simulink model "concept3_simulink_RL"  (R2025a)
settings: Solver=VariableStepAuto  StartTime=0.0  StopTime=Tf  FixedStep=0.001  MaxStep=0.01  MinStep=0.0001  RelTol=1e-3
InitFcn:
  | loaded_data = load('concept3_for_sim.mat');
  | robot = loaded_data.robot;
  | robot.DataFormat = 'column';
values from neighbouring files (symbols this model uses):
  mass = 40    [RL_main.m]    (also in baseline_sim.m)
  obs_vec = opa    [RL_main.m]    (also in baseline_sim.m)
  port = data(n, :)    [RL_main.m]    (also in baseline_sim.m = port_pos_data(n,:))
  port_num = 10    [RL_main.m]    (also in baseline_sim.m)
  port_target = AB2port(port_num)    [RL_main.m]    (also in baseline_sim.m)
  q0arm = rad2deg([-1.283; -1.622; 2.2761853; -1.8021853; 1.112; 1.859; 0.05328])    [RL_main.m]    (also in baseline_sim.m)
  q0b = [1; 0; 0; 0; 0; 0; 0]    [RL_main.m]    (also in baseline_sim.m = [1;0;0;0;0;0;0])
  sat_docked = AB2port(sat_docked_num)    [RL_main.m]    (also in baseline_sim.m)
  sat_docked_num = 6    [RL_main.m]    (also in baseline_sim.m)
  sim_state = 1    [RL_main.m]    (also in baseline_sim.m)
  Tlog = 0.1    [RL_main.m]    (also in baseline_sim.m)
  use_RL = 1    [RL_main.m]    (also in baseline_sim.m)
undefined symbols (not defined in the file or in its folder): opa, target, X, Y, Z
libraries: sm_lib x133, nesl_utility x67, simulink_extras x3, rllib x2
(part 5 of 6)

== matlab function concept3_simulink_RL/QP1/MATLAB Function2 ==
  data: ydot output; y output; done output; clock input; fromPort input; toPort input; seg output
function [ydot, y, done, seg] = Poly_traj_selector(clock, fromPort, toPort)
%#codegen
% Poly_traj_selector
% 입력:
%   - clock [s] : Simulink Clock 출력
%   - fromPort  : 시작 포트 번호 (uint8/uint16 권장)
%   - toPort    : 도착 포트 번호
%
% 출력:
%   - y = [x; y; z; roll; pitch; yaw] (deg for RPY)
%
% 설명:
% - 경로(포트쌍)별로 세그먼트 시간 T와 5차 다항 계수 coeffs를 등록해 둡니다.
% - 각 세그먼트는 정지/가속도0 경계조건을 만족하는 5차 다항 (열: [a5 a4 a3 a2 a1 a0]).
% - 세그먼트 개수는 예시로 3개(maxSeg=3)로 고정. (모자라면 뒤는 0초/0계수로 패딩)
% - 마지막 세그먼트 종료 이후에는 최종 자세를 홀드합니다.

% ===== 고정 파라미터 =====
maxSeg = int32(4);          % int32로 고정
nDOF   = int32(6);          % int32로 고정

% ===== 입력 포트 형 변환(내부는 int32 사용) =====
fromP = int32(fromPort);
toP   = int32(toPort);

% ===== 선택 키 (예: 6->10 = 610) =====
key = fromP*int32(100) + toP;

% ===== 메모리 미리 할당 (double) =====
T      = zeros(1, double(maxSeg));                % double
coeffs = zeros(double(nDOF), 6, double(maxSeg), 'like', clock);  % double
y      = zeros(double(nDOF), 1, 'like', clock);   % double
ydot   = zeros(double(nDOF), 1, 'like', clock);   % double
done = false;

switch key


    case 602
        % --- segment durations ---
        T1 = 47.987;
        T2 = 28;
        T3 = 20;
        T4 = 25;
        T  = [T1, T2, T3,T4];

        % --- coeffs(6,6,seg): rows=DOF [x y z roll pitch yaw], cols=[a5 a4 a3 a2 a1 a0] ---
        % Segment 1
        coeffs(:,:,1) = [ ...
 0	-0	 0	 0	 0	 2.5;
-3.18313416839e-08	 3.81874771732e-06	-0.000122167510444	 0	 0	 0.35;
 1.17893858088e-08	-1.41435100642e-06	 4.52472260904e-05	 0	 0	 0;
 0	-0	 0	 0	 0	-90;
 0	-0	 0	 0	 0	 0;
 0	-0	 0	 0	 0	-90

        ];

        % Segment 2
        coeffs(:,:,2) = [ ...
-4.88077884215e-07	 3.4165451895e-05	-0.000637755102041	 0	 0	 2.5;
 0	-0	 0	 0	 0	-1;
 0	-0	 0	 0	 0	 0.5;
 0	-0	 0	 0	 0	-90;
 0	-0	 0	 0	 0	 0;
 0	-0	 0	 0	 0	-90
        ];

        % Segment 3
        coeffs(:,:,3) = [ ...
 0	-0	 0	 0	 0	 1.1;
 0	-0	 0	 0	 0	-1;
 0	-0	 0	 0	 0	 0.5;
 0	-0	 0	 0	 0	-90;
 0	-0	 0	 0	 0	 0;
-0.00016875	 0.0084375	-0.1125	 0	 0	-90
        ];


        % Segment 4
        coeffs(:,:,4) = [ ...
 0	-0	 0	 0	 0	 1.1;
 0	-0	 0	 0	 0	-1;
-3.072e-07	 1.92e-05	-0.00032	 0	 0	 0.5;
 0	-0	 0	 0	 0	-90;
 0	-0	 0	 0	 0	 0;
 0	-0	 0	 0	 0	-180
        ];



 case 603
        % --- segment durations ---
        T1 = 47.987;
        T2 = 38;
        T3 = 20.0;
        T4 = 25;
        T  = [T1, T2, T3, T4];

        % --- coeffs(6,6,seg): rows=DOF [x y z roll pitch yaw], cols=[a5 a4 a3 a2 a1 a0] ---
        % Segment 1
        coeffs(:,:,1) = [ ...
 0	-0	 0	 0	 0	 2.5;
-3.18313416839e-08	 3.81874771732e-06	-0.000122167510444	 0	 0	 0.35;
 1.17893858088e-08	-1.41435100642e-06	 4.52472260904e-05	 0	 0	 0;
 0	-0	 0	 0	 0	-90;
 0	-0	 0	 0	 0	 0;
 0	-0	 0	 0	 0	-90
        ];

        % Segment 2
        coeffs(:,:,2) = [ ...
-1.43875507401e-07	 1.36681732031e-05	-0.000346260387812	 0	 0	 2.5;
 0	-0	 0	 0	 0	-1;
 0	-0	 0	 0	 0	 0.5;
 0	-0	 0	 0	 0	-90;
 0	-0	 0	 0	 0	 0;
 0	-0	 0	 0	 0	-90
        ];

        % Segment 3
        coeffs(:,:,3) = [ ...
 0	-0	 0	 0	 0	 0.6;
 0	-0	 0	 0	 0	-1;
 0	-0	 0	 0	 0	 0.5;
 0	-0	 0	 0	 0	-90;
 0	-0	 0	 0	 0	 0;
-0.00016875	 0.0084375	-0.1125	 0	 0	-90
        ];


        % Segment 4
        coeffs(:,:,4) = [ ...
 0	-0	 0	 0	 0	 0.6;
 0	-0	 0	 0	 0	-1;
-3.072e-07	 1.92e-05	-0.00032	 0	 0	 0.5;
 0	-0	 0	 0	 0	-90;
 0	-0	 0	 0	 0	 0;
 0	-0	 0	 0	 0	-180
        ];

    case 604
        % --- segment durations ---
        T1 = 47.987;
        T2 = 48;
        T3 = 20.0;
        T4 = 25;
        T  = [T1, T2, T3, T4];

        % --- coeffs(6,6,seg): rows=DOF [x y z roll pitch yaw], cols=[a5 a4 a3 a2 a1 a0] ---
        % Segment 1
        coeffs(:,:,1) = [ ...;
 0	-0	 0	 0	 0	 2.5;
-3.18313416839e-08	 3.81874771732e-06	-0.000122167510444	 0	 0	 0.35;
 1.17893858088e-08	-1.41435100642e-06	 4.52472260904e-05	 0	 0	 0;
 0	-0	 0	 0	 0	-90;
 0	-0	 0	 0	 0	 0;
 0	-0	 0	 0	 0	-90
        ];

        % Segment 2
        coeffs(:,:,2) = [ ...
-5.65140335648e-08	 6.78168402778e-06	-0.000217013888889	 0	 0	 2.5;
 0	-0	 0	 0	 0	-1;
 0	-0	 0	 0	 0	 0.5;
 0	-0	 0	 0	 0	-90;
 0	-0	 0	 0	 0	 0;
 0	-0	 0	 0	 0	-90
        ];

        % Segment 3
        coeffs(:,:,3) = [ ...
 0	-0	 0	 0	 0	 0.1;
 0	-0	 0	 0	 0	-1;
 0	-0	 0	 0	 0	 0.5;
 0	-0	 0	 0	 0	-90;
 0	-0	 0	 0	 0	 0;
-0.00016875	 0.0084375	-0.1125	 0	 0	-90
        ];

        % Segment 4
        coeffs(:,:,4) = [ ...
 0	-0	 0	 0	 0	 0.1;
 0	-0	 0	 0	 0	-1;
-3.072e-07	 1.92e-05	-0.00032	 0	 0	 0.5;
 0	-0	 0	 0	 0	-90;
 0	-0	 0	 0	 0	 0;
 0	-0	 0	 0	 0	-180
        ];


    case 605
        % --- segment durations ---
        T1 = 47.987;
        T2 = 58.000;
        T3 = 20;
        T4 = 25;
        T  = [T1, T2, T3, T4];

        % --- coeffs(6,6,seg): rows=DOF [x y z roll pitch yaw], cols=[a5 a4 a3 a2 a1 a0] ---
        % Segment 1
        coeffs(:,:,1) = [ ...;
 0	-0	 0	 0	 0	 2.5;
-3.18313416839e-08	 3.81874771732e-06	-0.000122167510444	 0	 0	 0.35;
 1.17893858088e-08	-1.41435100642e-06	 4.52472260904e-05	 0	 0	 0;
 0	-0	 0	 0	 0	-90;
 0	-0	 0	 0	 0	 0;
 0	-0	 0	 0	 0	-90
        ];

        % Segment 2
        coeffs(:,:,2) = [ ...
-2.65099726983e-08	 3.84394604125e-06	-0.000148632580262	 0	 0	 2.5;
 0	-0	 0	 0	 0	-1;
 0	-0	 0	 0	 0	 0.5;
 0	-0	 0	 0	 0	-90;
 0	-0	 0	 0	 0	 0;
 0	-0	 0	 0	 0	-90
        ];

        % Segment 3
        coeffs(:,:,3) = [ ...
 0	-0	 0	 0	 0	-0.4;
 0	-0	 0	 0	 0	-1;
 0	-0	 0	 0	 0	 0.5;
 0	-0	 0	 0	 0	-90;
 0	-0	 0	 0	 0	 0;
-0.00016875	 0.0084375	-0.1125	 0	 0	-90
        ];

        % Segment 4
        coeffs(:,:,4) = [ ...
 0	-0	 0	 0	 0	-0.4;
 0	-0	 0	 0	 0	-1;
-3.072e-07	 1.92e-05	-0.00032	 0	 0	 0.5;
 0	-0	 0	 0	 0	-90;
 0	-0	 0	 0	 0	 0;
 0	-0	 0	 0	 0	-180
        ];

    case 607
        % --- segment durations ---
        T1 = 27.335;
        T2 = 28.;
        T3 = 20;
        T4 = 25;
        T  = [T1, T2, T3,T4];

        % --- coeffs(6,6,seg): rows=DOF [x y z roll pitch yaw], cols=[a5 a4 a3 a2 a1 a0] ---
        % Segment 1
        coeffs(:,:,1) = [ ...
 0	-0	 0	 0	 0	 2.5;
 2.55528978563e-07	-1.74624452398e-05	 0.000318228218674	 0	 0	 0.35;
 1.96560752741e-07	-1.34326501845e-05	 0.000244790937442	 0	 0	 0;
 0	-0	 0	 0	 0	-90;
 0	-0	 0	 0	 0	 0;
 0	-0	 0	 0	 0	-90
        ];

        % Segment 2
        coeffs(:,:,2) = [ ...
-4.88077884215e-07	 3.4165451895e-05	-0.000637755102041	 0	 0	 2.5;
 0	-0	 0	 0	 0	 1;
 0	-0	 0	 0	 0	 0.5;
 0	-0	 0	 0	 0	-90;
 0	-0	 0	 0	 0	 0;
 0	-0	 0	 0	 0	-90
        ];

        % Segment 3
        coeffs(:,:,3) = [ ...
 0	-0	 0	 0	 0	 1.1;
 0	-0	 0	 0	 0	 1;
 0	-0	 0	 0	 0	 0.5;
 0	-0	 0	 0	 0	-90;
 0	-0	 0	 0	 0	 0;
 0.00016875	-0.0084375	 0.1125	 0	 0	-90
        ];

                % Segment 4
        coeffs(:,:,4) = [ ...
 0	-0	 0	 0	 0	 1.1;
 0	-0	 0	 0	 0	 1;
-3.072e-07	 1.92e-05	-0.00032	 0	 0	 0.5;
 0	-0	 0	 0	 0	-90;
 0	-0	 0	 0	 0	 0;
 0	-0	 0	 0	 0	 0
        ];

    case 608
        % --- segment durations ---
        T1 = 27.335;
        T2 = 38;
        T3 = 20;
        T4 = 25;
        T  = [T1, T2, T3,T4];

        % --- coeffs(6,6,seg): rows=DOF [x y z roll pitch yaw], cols=[a5 a4 a3 a2 a1 a0] ---
        % Segment 1
        coeffs(:,:,1) = [ ...
 0	-0	 0	 0	 0	 2.5;
 2.55528978563e-07	-1.74624452398e-05	 0.000318228218674	 0	 0	 0.35;
 1.96560752741e-07	-1.34326501845e-05	 0.000244790937442	 0	 0	 0;
 0	-0	 0	 0	 0	-90;
 0	-0	 0	 0	 0	 0;
 0	-0	 0	 0	 0	-90
        ];

        % Segment 2
        coeffs(:,:,2) = [ ...
-1.43875507401e-07	 1.36681732031e-05	-0.000346260387812	 0	 0	 2.5;
 0	-0	 0	 0	 0	 1;
 0	-0	 0	 0	 0	 0.5;
 0	-0	 0	 0	 0	-90;
 0	-0	 0	 0	 0	 0;
 0	-0	 0	 0	 0	-90
        ];

        % Segment 3
        coeffs(:,:,3) = [ ...
 0	-0	 0	 0	 0	 0.6;
 0	-0	 0	 0	 0	 1;
 0	-0	 0	 0	 0	 0.5;
 0	-0	 0	 0	 0	-90;
 0	-0	 0	 0	 0	 0;
 0.00016875	-0.0084375	 0.1125	 0	 0	-90

        ];

                % Segment 4
        coeffs(:,:,4) = [ ...
 0	-0	 0	 0	 0	 0.6;
 0	-0	 0	 0	 0	 1;
-3.072e-07	 1.92e-05	-0.00032	 0	 0	 0.5;
 0	-0	 0	 0	 0	-90;
 0	-0	 0	 0	 0	 0;
 0	-0	 0	 0	 0	 0
        ];
    
    case 609
        % --- segment durations ---
        T1 = 27.335;
        T2 = 48;
        T3 = 20;
        T4 = 25;
        T  = [T1, T2, T3, T4];

        % --- coeffs(6,6,seg): rows=DOF [x y z roll pitch yaw], cols=[a5 a4 a3 a2 a1 a0] ---
        % Segment 1
        coeffs(:,:,1) = [ ...
 0	-0	 0	 0	 0	 2.5;
 2.55528978563e-07	-1.74624452398e-05	 0.000318228218674	 0	 0	 0.35;
 1.96560752741e-07	-1.34326501845e-05	 0.000244790937442	 0	 0	 0;
 0	-0	 0	 0	 0	-90;
 0	-0	 0	 0	 0	 0;
 0	-0	 0	 0	 0	-90
        ];

        % Segment 2
        coeffs(:,:,2) = [ ...
-5.65140335648e-08	 6.78168402778e-06	-0.000217013888889	 0	 0	 2.5;
 0	-0	 0	 0	 0	 1;
 0	-0	 0	 0	 0	 0.5;
 0	-0	 0	 0	 0	-90;
 0	-0	 0	 0	 0	 0;
 0	-0	 0	 0	 0	-90
        ];

        % Segment 3
        coeffs(:,:,3) = [ ...
 0	-0	 0	 0	 0	 0.1;
 0	-0	 0	 0	 0	 1;
 0	-0	 0	 0	 0	 0.5;
 0	-0	 0	 0	 0	-90;
 0	-0	 0	 0	 0	 0;
 0.00016875	-0.0084375	 0.1125	 0	 0	-90
        ];

        % Segment 4
        coeffs(:,:,4) = [ ...
 0	-0	 0	 0	 0	 0.1;
 0	-0	 0	 0	 0	 1;
-3.072e-07	 1.92e-05	-0.00032	 0	 0	 0.5;
 0	-0	 0	 0	 0	-90;
 0	-0	 0	 0	 0	 0;
 0	-0	 0	 0	 0	 0
        ];
%{
%더 위로 많이 튀어오루는
 case 610
        % --- segment durations ---
        T1 = 34.359;
        T2 = 58.000;
        T3 = 20.0;
        T4 = 40.0;
        T  = [T1, T2, T3,T4];

        % --- coeffs(6,6,seg): rows=DOF [x y z roll pitch yaw], cols=[a5 a4 a3 a2 a1 a0] ---
        % Segment 1
        coeffs(:,:,1) = [ ...
 0	-0	 0	 0	 0	 2.5;
 8.14420194226e-08	-6.99570934256e-06	 0.000160244714142	 0	 0	 0.35;
 1.00236331597e-07	-8.61010380623e-06	 0.000197224263559	 0	 0	 0;
 0	-0	 0	 0	 0	-90;
 0	-0	 0	 0	 0	 0;
 0	-0	 0	 0	 0	-90
        ];

        % Segment 2
        coeffs(:,:,2) = [ ...
-2.65099726983e-08	 3.84394604125e-06	-0.000148632580262	 0	 0	 2.5;
 0	-0	 0	 0	 0	 1;
 0	-0	 0	 0	 0	 0.8;
 0	-0	 0	 0	 0	-90;
 0	-0	 0	 0	 0	 0;
 0	-0	 0	 0	 0	-90
        ];

        % Segment 3
        coeffs(:,:,3) = [ ...
 0	-0	 0	 0	 0	-0.4;
 0	-0	 0	 0	 0	 1;
 0	-0	 0	 0	 0	 0.8;
 0	-0	 0	 0	 0	-90;
 0	-0	 0	 0	 0	 0;
 0.00016875	-0.0084375	 0.1125	 0	 0	-90
        ];

        % Segment 4
        coeffs(:,:,4) = [ ...
 0	-0	 0	 0	 0	-0.4;
 0	-0	 0	 0	 0	 1;
-4.6875e-08	 4.6875e-06	-0.000125	 0	 0	 0.8;
 0	-0	 0	 0	 0	-90;
 0	-0	 0	 0	 0	 0;
 0	-0	 0	 0	 0	 0
        ];
%}


    case 610
        % --- segment durations ---
        T1 = 32.8718048721934 ;
        T2 = 58.000;
        T3 = 20.0;
        T4 = 26.9258240356725;
        T  = [T1, T2, T3,T4];

        % --- coeffs(6,6,seg): rows=DOF [x y z roll pitch yaw], cols=[a5 a4 a3 a2 a1 a0] ---
        % Segment 1
        coeffs(:,:,1) = [ ...
 0	-0	 0	 0	 0	 2.5;
 1.32877798661e-07	-1.09198326736e-05	 0.000239303072589	 0	 0	 0.35;
 7.81634109771e-08	-6.42343098446e-06	 0.000140766513288	 0	 0	 0;
 0	-0	 0	 0	 0	-90;
 0	-0	 0	 0	 0	 0;
 0	-0	 0	 0	 0	-90
        ];

        % Segment 2
        coeffs(:,:,2) = [ ...
-2.65099726983e-08	 3.84394604125e-06	-0.000148632580262	 0	 0	 2.5;
 0	-0	 0	 0	 0	 1.2;
 0	-0	 0	 0	 0	 0.5;
 0	-0	 0	 0	 0	-90;
 0	-0	 0	 0	 0	 0;
 0	-0	 0	 0	 0	-90
        ];

        % Segment 3
        coeffs(:,:,3) = [ ...
 0	-0	 0	 0	 0	-0.4;
 0	-0	 0	 0	 0	 1.2;
 0	-0	 0	 0	 0	 0.5;
 0	-0	 0	 0	 0	-90;
 0	-0	 0	 0	 0	 0;
 0.00016875	-0.0084375	 0.1125	 0	 0	-90
        ];

        % Segment 4
        coeffs(:,:,4) = [ ...
 0	-0	 0	 0	 0	-0.4;
-8.47883589298e-08	 5.70749108205e-06	-0.000102452600374	 0	 0	 1.2;
-2.11970897325e-07	 1.42687277051e-05	-0.000256131500934	 0	 0	 0.5;
 0	-0	 0	 0	 0	-90;
 0	-0	 0	 0	 0	 0;
 0	-0	 0	 0	 0	 0
        ];

        
    % =========================



    otherwise
        seg = double(0);
        return;
end
% ===== 누적 시간 & 세그먼트 선택(모두 int32 사용) =====
cumT = zeros(1, double(maxSeg));
cumT(1) = T(1);
for i = 2:double(maxSeg)
    cumT(i) = cumT(i-1) + T(i);
end

t = clock;
seg_i = int32(1);
t0 = 0.0;

% ===== 현재 세그먼트 판별 =====
if t <= 0
    seg_i = int32(1); t0 = 0.0;
else
    lastSeg = int32(1);
    for i = int32(1):maxSeg
        if T(double(i)) > 0
            lastSeg = i;
        end
    end

    if t < cumT(1)
        seg_i = int32(1); t0 = 0.0;
    elseif (maxSeg >= 2) && (T(2) > 0) && (t < cumT(2))
        seg_i = int32(2); t0 = cumT(1);
    elseif (maxSeg >= 3) && (T(3) > 0) && (t < cumT(3))
        seg_i = int32(3); t0 = cumT(2);
    elseif (maxSeg >= 4) && (T(4) > 0) && (t < cumT(4))
        seg_i = int32(4); t0 = cumT(3);
    else
        seg_i = lastSeg;
        if lastSeg == 1
            t0 = 0.0;
        else
            t0 = cumT(double(lastSeg-1));
        end
        t = cumT(double(lastSeg)); % clamp
        done = true;
    end
end

% ===== 현재 세그먼트 double로 변환해 출력용 저장 =====
seg = double(seg_i);

% ===== 세그먼트 상대시간 =====
tau = t - t0;

% ===== Horner 평가 =====
for d = 1:double(nDOF)
    a5 = coeffs(d,1,seg_i);
    a4 = coeffs(d,2,seg_i);
    a3 = coeffs(d,3,seg_i);
    a2 = coeffs(d,4,seg_i);
    a1 = coeffs(d,5,seg_i);
    a0 = coeffs(d,6,seg_i);
    y(d)    = ((((a5*tau + a4)*tau + a3)*tau + a2)*tau + a1)*tau + a0;
    ydot(d) = ((((5*a5*tau + 4*a4)*tau + 3*a3)*tau + 2*a2)*tau + a1);
end
ydot(4:6) = deg2rad(ydot(4:6));
%y(3) = 0;
%ydot(3) = 0;
end

== matlab function concept3_simulink_RL/R2L/obs ==
  data: q input; y output; qdot input; w_base input; Tau input; H_obs input; muRL input; sigmaRL input; muRL_new output; sigmaRL_new output
function [y, muRL_new, sigmaRL_new] = obs(q, qdot, w_base, Tau, H_obs, muRL, sigmaRL)
%% --------------------------------------------------------------
% q : [quat_base(4); basepos(3); joint(7)]  (14x1)
% qdot : (7x1)
% H_obs : RL_obs 벡터 (26x1)
% muRL, sigmaRL : 이전 호출의 통계량 (26x1)
% --------------------------------------------------------------
eps = 1e-8;
beta = 0.05;

%% (1) 입력 분리
qbase = q(1:4);
q_joint = q(8:14);

%% (2) 관절 각도/속도 정규화
q_min = [-1.3 -2.9 2.2 -2.8 1.1 1.3 0.1]';
q_max = [2.2 -1.6 4.4 -1.5 3.9 4.4 2.1]';
qdot_max = [0.2 0.07 0.1 0.08 0.23 0.1 0.08]';

q_mid = 0.5 * (q_max + q_min);
q_norm = 2 * (q_joint - q_mid) ./ (q_max - q_min);
qdot_norm = qdot ./ (qdot_max + eps);
qdot_norm = max(min(qdot_norm, 1), -1);

%% (3) 베이스 쿼터니언 정규화
q_base = qbase / (norm(qbase) + eps);   % 정규화
if q_base(1) < 0, q_base = -q_base; end % 연속성 확보

q_ref = [1;0;0;0];                      % 목표자세
q_err = quatmultiply(q_ref.', quatconj(q_base.')).';  % [w x y z]

if q_err(1) < 0, q_err = -q_err; end    % 부호 연속성

att_err_vec = 2 * q_err(2:4);
qbase = att_err_vec / deg2rad(20);   % 약 [-1,1] 범위로 정규화


%% 베이스 속도 정규화
qb_max = 0.004; qb_min = -0.004;
qb_mid = 0.5 * (qb_max + qb_min);
qb_norm = 2 * (w_base - qb_mid) ./ (qb_max - qb_min);

%% 토크 정규화
t_max = 3; t_min = -3;
t_mid = 0.5 * (t_max + t_min);
t_norm = 2 * (Tau - t_mid) ./ (t_max - t_min);

%% (4) RL_obs 정규화
RL_obs = H_obs(:);
RL_log = sign(RL_obs) .* log(1 + abs(RL_obs));

% 입력된 muRL, sigmaRL이 없으면 기본값 세팅
if isempty(muRL)
    muRL = zeros(size(RL_obs));
    sigmaRL = ones(size(RL_obs));
end

% 러닝 평균 갱신
muRL_new    = (1 - beta) * muRL + beta * RL_log;
sigmaRL_new = (1 - beta) * sigmaRL + beta * abs(RL_log - muRL_new);

% 정규화 및 클리핑
RL_norm = (RL_log - muRL_new) ./ (sigmaRL_new + eps);
RL_norm = max(min(RL_norm, 5), -5);

% RL_norm 빼면 18

%% (5) 출력 구성

%y = [q_norm; qdot_norm; qbase; qb_norm; t_norm; RL_norm];
y = [q_norm; qdot_norm; t_norm];
end

== matlab function concept3_simulink_RL/Plant/Docking logic/Docking sensor/Subsystem/Quat2RPY ==
  data: q_current input; RPY output
function RPY = fcn(q_current)

sequence = 'ZYX';

eul_angles_rad_out = quat2eul(q_current', sequence);

%eul_angles_deg_out = rad2deg(eul_angles_rad_out);

yaw_out = eul_angles_rad_out(1);
pitch_out = eul_angles_rad_out(2);
roll_out = eul_angles_rad_out(3);

RPY = [roll_out; pitch_out; yaw_out];

== matlab function concept3_simulink_RL/Plant/station_robot_arm/Subsystem/Quat2RPY ==
  data: q_current input; RPY output
function RPY = fcn(q_current)

sequence = 'ZYX';

eul_angles_rad_out = quat2eul(q_current', sequence);

eul_angles_deg_out = rad2deg(eul_angles_rad_out);

yaw_deg_out = eul_angles_deg_out(1);
pitch_deg_out = eul_angles_deg_out(2);
roll_deg_out = eul_angles_deg_out(3);

RPY = [roll_deg_out; pitch_deg_out; yaw_deg_out];

== matlab function concept3_simulink_RL/R2L/MATLAB Function1 ==
  data: xb_q input; w_base input; tau input; r output
function r = reward_fn(xb_q,w_base, tau)
%#codegen
% RL 보상함수 (exponential terminal shaping)
% xb_q : [quat(4); pos(3)]
% q : full state (joint 포함)
% tau : joint torque
% done : episode 종료 flag

%% ====== 가중치 설정 ======
alpha = 0.3;    % 조인트 복귀 가중치
beta  = 20000.0;    % 베이스 각속도
gamma = 200;     % 토크 절약 가중치
delta = 150;   % 베이스 자세 오차 가중치

offset = 0.0;     % baseline offset (critic 안정화용)
scale = 1;      % 전체 보상 스케일 조절

%% ====== 데이터 정리 ======
xb_q = double(xb_q(:));
%q    = double(q(:));
tau  = double(tau(:));
w_base = double(w_base(:));
k_att = 1.0;

%% ====== (1) 조인트각 오차 ======
%{
qhome = deg2rad([-90; -90; 150; -120; 60; -90; 0]);
joint_err = qhome - q(8:14);
joint_err_norm = sqrt(mean(joint_err.^2));   % rad

% --- 0~1 정규화 ---
q_norm = min(joint_err_norm / deg2rad(180), 1.0);  % 180° 기준
joint_term = alpha * q_norm^2;
%}
%% ====== (2) 토크 절약 항 ======
tau_norm = min(sum(tau.^2) / (50^2), 1.0);   % 대략 50 N·m 기준
torque_term = gamma * tau_norm;
torque_term = min(torque_term,1);
%torque_term = 0;
%% ====== (3) 베이스 자세 오차 ======
q_base = xb_q(1:4);  
q_base = q_base / (norm(q_base)+1e-12);
q_ref  = [1;0;0;0];

q_rel_w = abs(q_ref(1)*q_base(1) + dot(q_ref(2:4), q_base(2:4)));
q_rel_v = q_base(2:4);
angle_diff = 2*atan2(norm(q_rel_v), max(q_rel_w, 1e-12)); % rad

att_norm = min(angle_diff / pi, 1.0);    % 최대 π rad (=180°)
att_sharp = 1 - exp(-5 * (att_norm / deg2rad(3))^2);  % 0.26rad≈15°, 감도조정
%base_att_term = delta * att_sharp;
base_att_term = delta * att_norm^2;
%base_att_term = min(base_att_term,1);
%% --- (4) 베이스 회전속도 억제 ---
base_rot_term = beta * sum(w_base.^2);
base_rot_term = min(base_rot_term,1);

%% ====== (4) Step reward (정규화 + offset) ======
raw_step = -(base_att_term + 0.5*torque_term + base_rot_term);
step_reward = scale * (raw_step + offset);   % offset 적용

%% ====== (6) 총 보상 ======
%r = step_reward;
r = [ base_att_term  torque_term  base_rot_term];
%r = max(min(r, +1000), -1000);  % 클리핑W
end

== matlab function concept3_simulink_RL/QP1/MATLAB Function3 ==
  data: u input; y output
function y = fcn(u)

y = u(1:3,4);

== matlab function concept3_simulink_RL/Plant/station_robot_arm/MATLAB Function1 ==
  data: R input; T_ab2dp output; p input
function T_ab2dp = fcn(R,p)

T_ab2dp = [R,p;0 0 0 1];

== matlab function concept3_simulink_RL/QP1/MATLAB Function4 ==
  data: ydot output; y output; done output; clock input; fromPort input; toPort input; seg output
function [ydot, y, done, seg] = Poly_traj_selector(clock, fromPort, toPort)
%#codegen
% Poly_traj_selector
% 입력:
%   - clock [s] : Simulink Clock 출력
%   - fromPort  : 시작 포트 번호 (uint8/uint16 권장)
%   - toPort    : 도착 포트 번호
%
% 출력:
%   - y = [x; y; z; roll; pitch; yaw] (deg for RPY)
%
% 설명:
% - 경로(포트쌍)별로 세그먼트 시간 T와 5차 다항 계수 coeffs를 등록해 둡니다.
% - 각 세그먼트는 정지/가속도0 경계조건을 만족하는 5차 다항 (열: [a5 a4 a3 a2 a1 a0]).
% - 세그먼트 개수는 예시로 3개(maxSeg=3)로 고정. (모자라면 뒤는 0초/0계수로 패딩)
% - 마지막 세그먼트 종료 이후에는 최종 자세를 홀드합니다.

% ===== 고정 파라미터 =====
maxSeg = int32(4);          % int32로 고정
nDOF   = int32(6);          % int32로 고정

% ===== 입력 포트 형 변환(내부는 int32 사용) =====
fromP = int32(fromPort);
toP   = int32(toPort);

% ===== 선택 키 (예: 6->10 = 610) =====
key = fromP*int32(100) + toP;

% ===== 메모리 미리 할당 (double) =====
T      = zeros(1, double(maxSeg));                % double
coeffs = zeros(double(nDOF), 6, double(maxSeg), 'like', clock);  % double
y      = zeros(double(nDOF), 1, 'like', clock);   % double
ydot   = zeros(double(nDOF), 1, 'like', clock);   % double
done = false;

switch key


    case 602
        % --- segment durations ---
        T1 = 47.987;
        T2 = 28;
        T3 = 20;
        T4 = 25;
        T  = [T1, T2, T3,T4];

        % --- coeffs(6,6,seg): rows=DOF [x y z roll pitch yaw], cols=[a5 a4 a3 a2 a1 a0] ---
        % Segment 1
        coeffs(:,:,1) = [ ...
 0	-0	 0	 0	 0	 2.5;
-3.18313416839e-08	 3.81874771732e-06	-0.000122167510444	 0	 0	 0.35;
 1.17893858088e-08	-1.41435100642e-06	 4.52472260904e-05	 0	 0	 0;
 0	-0	 0	 0	 0	-90;
 0	-0	 0	 0	 0	 0;
 0	-0	 0	 0	 0	-90

        ];

        % Segment 2
        coeffs(:,:,2) = [ ...
-4.88077884215e-07	 3.4165451895e-05	-0.000637755102041	 0	 0	 2.5;
 0	-0	 0	 0	 0	-1;
 0	-0	 0	 0	 0	 0.5;
 0	-0	 0	 0	 0	-90;
 0	-0	 0	 0	 0	 0;
 0	-0	 0	 0	 0	-90
        ];

        % Segment 3
        coeffs(:,:,3) = [ ...
 0	-0	 0	 0	 0	 1.1;
 0	-0	 0	 0	 0	-1;
 0	-0	 0	 0	 0	 0.5;
 0	-0	 0	 0	 0	-90;
 0	-0	 0	 0	 0	 0;
-0.00016875	 0.0084375	-0.1125	 0	 0	-90
        ];


        % Segment 4
        coeffs(:,:,4) = [ ...
 0	-0	 0	 0	 0	 1.1;
 0	-0	 0	 0	 0	-1;
-3.072e-07	 1.92e-05	-0.00032	 0	 0	 0.5;
 0	-0	 0	 0	 0	-90;
 0	-0	 0	 0	 0	 0;
 0	-0	 0	 0	 0	-180
        ];



 case 603
        % --- segment durations ---
        T1 = 47.987;
        T2 = 38;
        T3 = 20.0;
        T4 = 25;
        T  = [T1, T2, T3, T4];

        % --- coeffs(6,6,seg): rows=DOF [x y z roll pitch yaw], cols=[a5 a4 a3 a2 a1 a0] ---
        % Segment 1
        coeffs(:,:,1) = [ ...
 0	-0	 0	 0	 0	 2.5;
-3.18313416839e-08	 3.81874771732e-06	-0.000122167510444	 0	 0	 0.35;
 1.17893858088e-08	-1.41435100642e-06	 4.52472260904e-05	 0	 0	 0;
 0	-0	 0	 0	 0	-90;
 0	-0	 0	 0	 0	 0;
 0	-0	 0	 0	 0	-90
        ];

        % Segment 2
        coeffs(:,:,2) = [ ...
-1.43875507401e-07	 1.36681732031e-05	-0.000346260387812	 0	 0	 2.5;
 0	-0	 0	 0	 0	-1;
 0	-0	 0	 0	 0	 0.5;
 0	-0	 0	 0	 0	-90;
 0	-0	 0	 0	 0	 0;
 0	-0	 0	 0	 0	-90
        ];

        % Segment 3
        coeffs(:,:,3) = [ ...
 0	-0	 0	 0	 0	 0.6;
 0	-0	 0	 0	 0	-1;
 0	-0	 0	 0	 0	 0.5;
 0	-0	 0	 0	 0	-90;
 0	-0	 0	 0	 0	 0;
-0.00016875	 0.0084375	-0.1125	 0	 0	-90
        ];


        % Segment 4
        coeffs(:,:,4) = [ ...
 0	-0	 0	 0	 0	 0.6;
 0	-0	 0	 0	 0	-1;
-3.072e-07	 1.92e-05	-0.00032	 0	 0	 0.5;
 0	-0	 0	 0	 0	-90;
 0	-0	 0	 0	 0	 0;
 0	-0	 0	 0	 0	-180
        ];

    case 604
        % --- segment durations ---
        T1 = 47.987;
        T2 = 48;
        T3 = 20.0;
        T4 = 25;
        T  = [T1, T2, T3, T4];

        % --- coeffs(6,6,seg): rows=DOF [x y z roll pitch yaw], cols=[a5 a4 a3 a2 a1 a0] ---
        % Segment 1
        coeffs(:,:,1) = [ ...;
 0	-0	 0	 0	 0	 2.5;
-3.18313416839e-08	 3.81874771732e-06	-0.000122167510444	 0	 0	 0.35;
 1.17893858088e-08	-1.41435100642e-06	 4.52472260904e-05	 0	 0	 0;
 0	-0	 0	 0	 0	-90;
 0	-0	 0	 0	 0	 0;
 0	-0	 0	 0	 0	-90
        ];

        % Segment 2
        coeffs(:,:,2) = [ ...
-5.65140335648e-08	 6.78168402778e-06	-0.000217013888889	 0	 0	 2.5;
 0	-0	 0	 0	 0	-1;
 0	-0	 0	 0	 0	 0.5;
 0	-0	 0	 0	 0	-90;
 0	-0	 0	 0	 0	 0;
 0	-0	 0	 0	 0	-90
        ];

        % Segment 3
        coeffs(:,:,3) = [ ...
 0	-0	 0	 0	 0	 0.1;
 0	-0	 0	 0	 0	-1;
 0	-0	 0	 0	 0	 0.5;
 0	-0	 0	 0	 0	-90;
 0	-0	 0	 0	 0	 0;
-0.00016875	 0.0084375	-0.1125	 0	 0	-90
        ];

        % Segment 4
        coeffs(:,:,4) = [ ...
 0	-0	 0	 0	 0	 0.1;
 0	-0	 0	 0	 0	-1;
-3.072e-07	 1.92e-05	-0.00032	 0	 0	 0.5;
 0	-0	 0	 0	 0	-90;
 0	-0	 0	 0	 0	 0;
 0	-0	 0	 0	 0	-180
        ];


    case 605
        % --- segment durations ---
        T1 = 47.987;
        T2 = 58.000;
        T3 = 20;
        T4 = 25;
        T  = [T1, T2, T3, T4];

        % --- coeffs(6,6,seg): rows=DOF [x y z roll pitch yaw], cols=[a5 a4 a3 a2 a1 a0] ---
        % Segment 1
        coeffs(:,:,1) = [ ...;
 0	-0	 0	 0	 0	 2.5;
-3.18313416839e-08	 3.81874771732e-06	-0.000122167510444	 0	 0	 0.35;
 1.17893858088e-08	-1.41435100642e-06	 4.52472260904e-05	 0	 0	 0;
 0	-0	 0	 0	 0	-90;
 0	-0	 0	 0	 0	 0;
 0	-0	 0	 0	 0	-90
        ];

        % Segment 2
        coeffs(:,:,2) = [ ...
-2.65099726983e-08	 3.84394604125e-06	-0.000148632580262	 0	 0	 2.5;
 0	-0	 0	 0	 0	-1;
 0	-0	 0	 0	 0	 0.5;
 0	-0	 0	 0	 0	-90;
 0	-0	 0	 0	 0	 0;
 0	-0	 0	 0	 0	-90
        ];

        % Segment 3
        coeffs(:,:,3) = [ ...
 0	-0	 0	 0	 0	-0.4;
 0	-0	 0	 0	 0	-1;
 0	-0	 0	 0	 0	 0.5;
 0	-0	 0	 0	 0	-90;
 0	-0	 0	 0	 0	 0;
-0.00016875	 0.0084375	-0.1125	 0	 0	-90
        ];

        % Segment 4
        coeffs(:,:,4) = [ ...
 0	-0	 0	 0	 0	-0.4;
 0	-0	 0	 0	 0	-1;
-3.072e-07	 1.92e-05	-0.00032	 0	 0	 0.5;
 0	-0	 0	 0	 0	-90;
 0	-0	 0	 0	 0	 0;
 0	-0	 0	 0	 0	-180
        ];

    case 607
        % --- segment durations ---
        T1 = 27.335;
        T2 = 28.;
        T3 = 20;
        T4 = 25;
        T  = [T1, T2, T3,T4];

        % --- coeffs(6,6,seg): rows=DOF [x y z roll pitch yaw], cols=[a5 a4 a3 a2 a1 a0] ---
        % Segment 1
        coeffs(:,:,1) = [ ...
 0	-0	 0	 0	 0	 2.5;
 2.55528978563e-07	-1.74624452398e-05	 0.000318228218674	 0	 0	 0.35;
 1.96560752741e-07	-1.34326501845e-05	 0.000244790937442	 0	 0	 0;
 0	-0	 0	 0	 0	-90;
 0	-0	 0	 0	 0	 0;
 0	-0	 0	 0	 0	-90
        ];

        % Segment 2
        coeffs(:,:,2) = [ ...
-4.88077884215e-07	 3.4165451895e-05	-0.000637755102041	 0	 0	 2.5;
 0	-0	 0	 0	 0	 1;
 0	-0	 0	 0	 0	 0.5;
 0	-0	 0	 0	 0	-90;
 0	-0	 0	 0	 0	 0;
 0	-0	 0	 0	 0	-90
        ];

        % Segment 3
        coeffs(:,:,3) = [ ...
 0	-0	 0	 0	 0	 1.1;
 0	-0	 0	 0	 0	 1;
 0	-0	 0	 0	 0	 0.5;
 0	-0	 0	 0	 0	-90;
 0	-0	 0	 0	 0	 0;
 0.00016875	-0.0084375	 0.1125	 0	 0	-90
        ];

                % Segment 4
        coeffs(:,:,4) = [ ...
 0	-0	 0	 0	 0	 1.1;
 0	-0	 0	 0	 0	 1;
-3.072e-07	 1.92e-05	-0.00032	 0	 0	 0.5;
 0	-0	 0	 0	 0	-90;
 0	-0	 0	 0	 0	 0;
 0	-0	 0	 0	 0	 0
        ];

    case 608
        % --- segment durations ---
        T1 = 27.335;
        T2 = 38;
        T3 = 20;
        T4 = 25;
        T  = [T1, T2, T3,T4];

        % --- coeffs(6,6,seg): rows=DOF [x y z roll pitch yaw], cols=[a5 a4 a3 a2 a1 a0] ---
        % Segment 1
        coeffs(:,:,1) = [ ...
 0	-0	 0	 0	 0	 2.5;
 2.55528978563e-07	-1.74624452398e-05	 0.000318228218674	 0	 0	 0.35;
 1.96560752741e-07	-1.34326501845e-05	 0.000244790937442	 0	 0	 0;
 0	-0	 0	 0	 0	-90;
 0	-0	 0	 0	 0	 0;
 0	-0	 0	 0	 0	-90
        ];

        % Segment 2
        coeffs(:,:,2) = [ ...
-1.43875507401e-07	 1.36681732031e-05	-0.000346260387812	 0	 0	 2.5;
 0	-0	 0	 0	 0	 1;
 0	-0	 0	 0	 0	 0.5;
 0	-0	 0	 0	 0	-90;
 0	-0	 0	 0	 0	 0;
 0	-0	 0	 0	 0	-90
        ];

        % Segment 3
        coeffs(:,:,3) = [ ...
 0	-0	 0	 0	 0	 0.6;
 0	-0	 0	 0	 0	 1;
 0	-0	 0	 0	 0	 0.5;
 0	-0	 0	 0	 0	-90;
 0	-0	 0	 0	 0	 0;
 0.00016875	-0.0084375	 0.1125	 0	 0	-90

        ];

                % Segment 4
        coeffs(:,:,4) = [ ...
 0	-0	 0	 0	 0	 0.6;
 0	-0	 0	 0	 0	 1;
-3.072e-07	 1.92e-05	-0.00032	 0	 0	 0.5;
 0	-0	 0	 0	 0	-90;
 0	-0	 0	 0	 0	 0;
 0	-0	 0	 0	 0	 0
        ];
    
    case 609
        % --- segment durations ---
        T1 = 27.335;
        T2 = 48;
        T3 = 20;
        T4 = 25;
        T  = [T1, T2, T3, T4];

        % --- coeffs(6,6,seg): rows=DOF [x y z roll pitch yaw], cols=[a5 a4 a3 a2 a1 a0] ---
        % Segment 1
        coeffs(:,:,1) = [ ...
 0	-0	 0	 0	 0	 2.5;
 2.55528978563e-07	-1.74624452398e-05	 0.000318228218674	 0	 0	 0.35;
 1.96560752741e-07	-1.34326501845e-05	 0.000244790937442	 0	 0	 0;
 0	-0	 0	 0	 0	-90;
 0	-0	 0	 0	 0	 0;
 0	-0	 0	 0	 0	-90
        ];

        % Segment 2
        coeffs(:,:,2) = [ ...
-5.65140335648e-08	 6.78168402778e-06	-0.000217013888889	 0	 0	 2.5;
 0	-0	 0	 0	 0	 1;
 0	-0	 0	 0	 0	 0.5;
 0	-0	 0	 0	 0	-90;
 0	-0	 0	 0	 0	 0;
 0	-0	 0	 0	 0	-90
        ];

        % Segment 3
        coeffs(:,:,3) = [ ...
 0	-0	 0	 0	 0	 0.1;
 0	-0	 0	 0	 0	 1;
 0	-0	 0	 0	 0	 0.5;
 0	-0	 0	 0	 0	-90;
 0	-0	 0	 0	 0	 0;
 0.00016875	-0.0084375	 0.1125	 0	 0	-90
        ];

        % Segment 4
        coeffs(:,:,4) = [ ...
 0	-0	 0	 0	 0	 0.1;
 0	-0	 0	 0	 0	 1;
-3.072e-07	 1.92e-05	-0.00032	 0	 0	 0.5;
 0	-0	 0	 0	 0	-90;
 0	-0	 0	 0	 0	 0;
 0	-0	 0	 0	 0	 0
        ];
%{
%더 위로 많이 튀어오루는
 case 610
        % --- segment durations ---
        T1 = 34.359;
        T2 = 58.000;
        T3 = 20.0;
        T4 = 40.0;
        T  = [T1, T2, T3,T4];

        % --- coeffs(6,6,seg): rows=DOF [x y z roll pitch yaw], cols=[a5 a4 a3 a2 a1 a0] ---
        % Segment 1
        coeffs(:,:,1) = [ ...
 0	-0	 0	 0	 0	 2.5;
 8.14420194226e-08	-6.99570934256e-06	 0.000160244714142	 0	 0	 0.35;
 1.00236331597e-07	-8.61010380623e-06	 0.000197224263559	 0	 0	 0;
 0	-0	 0	 0	 0	-90;
 0	-0	 0	 0	 0	 0;
 0	-0	 0	 0	 0	-90
        ];

        % Segment 2
        coeffs(:,:,2) = [ ...
-2.65099726983e-08	 3.84394604125e-06	-0.000148632580262	 0	 0	 2.5;
 0	-0	 0	 0	 0	 1;
 0	-0	 0	 0	 0	 0.8;
 0	-0	 0	 0	 0	-90;
 0	-0	 0	 0	 0	 0;
 0	-0	 0	 0	 0	-90
        ];

        % Segment 3
        coeffs(:,:,3) = [ ...
 0	-0	 0	 0	 0	-0.4;
 0	-0	 0	 0	 0	 1;
 0	-0	 0	 0	 0	 0.8;
 0	-0	 0	 0	 0	-90;
 0	-0	 0	 0	 0	 0;
 0.00016875	-0.0084375	 0.1125	 0	 0	-90
        ];

        % Segment 4
        coeffs(:,:,4) = [ ...
 0	-0	 0	 0	 0	-0.4;
 0	-0	 0	 0	 0	 1;
-4.6875e-08	 4.6875e-06	-0.000125	 0	 0	 0.8;
 0	-0	 0	 0	 0	-90;
 0	-0	 0	 0	 0	 0;
 0	-0	 0	 0	 0	 0
        ];
%}


    case 610
        % --- segment durations ---
        T1 = 32.8718048721934 ;
        T2 = 58.000;
        T3 = 20.0;
        T4 = 26.9258240356725;
        T  = [T1, T2, T3,T4];

        % --- coeffs(6,6,seg): rows=DOF [x y z roll pitch yaw], cols=[a5 a4 a3 a2 a1 a0] ---
        % Segment 1
        coeffs(:,:,1) = [ ...
 0	-0	 0	 0	 0	 2.5;
 1.32877798661e-07	-1.09198326736e-05	 0.000239303072589	 0	 0	 0.35;
 7.81634109771e-08	-6.42343098446e-06	 0.000140766513288	 0	 0	 0;
 0	-0	 0	 0	 0	-90;
 0	-0	 0	 0	 0	 0;
 0	-0	 0	 0	 0	-90
        ];

        % Segment 2
        coeffs(:,:,2) = [ ...
-2.65099726983e-08	 3.84394604125e-06	-0.000148632580262	 0	 0	 2.5;
 0	-0	 0	 0	 0	 1.2;
 0	-0	 0	 0	 0	 0.5;
 0	-0	 0	 0	 0	-90;
 0	-0	 0	 0	 0	 0;
 0	-0	 0	 0	 0	-90
        ];

        % Segment 3
        coeffs(:,:,3) = [ ...
 0	-0	 0	 0	 0	-0.4;
 0	-0	 0	 0	 0	 1.2;
 0	-0	 0	 0	 0	 0.5;
 0	-0	 0	 0	 0	-90;
 0	-0	 0	 0	 0	 0;
 0.00016875	-0.0084375	 0.1125	 0	 0	-90
        ];

        % Segment 4
        coeffs(:,:,4) = [ ...
 0	-0	 0	 0	 0	-0.4;
-8.47883589298e-08	 5.70749108205e-06	-0.000102452600374	 0	 0	 1.2;
-2.11970897325e-07	 1.42687277051e-05	-0.000256131500934	 0	 0	 0.5;
 0	-0	 0	 0	 0	-90;
 0	-0	 0	 0	 0	 0;
 0	-0	 0	 0	 0	 0
        ];

        
    % =========================



    otherwise
        seg = double(0);
        return;
end
% ===== 누적 시간 & 세그먼트 선택(모두 int32 사용) =====
cumT = zeros(1, double(maxSeg));
cumT(1) = T(1);
for i = 2:double(maxSeg)
    cumT(i) = cumT(i-1) + T(i);
end

t = clock;
seg_i = int32(1);
t0 = 0.0;

% ===== 현재 세그먼트 판별 =====
if t <= 0
    seg_i = int32(1); t0 = 0.0;
else
    lastSeg = int32(1);
    for i = int32(1):maxSeg
        if T(double(i)) > 0
            lastSeg = i;
        end
    end

    if t < cumT(1)
        seg_i = int32(1); t0 = 0.0;
    elseif (maxSeg >= 2) && (T(2) > 0) && (t < cumT(2))
        seg_i = int32(2); t0 = cumT(1);
    elseif (maxSeg >= 3) && (T(3) > 0) && (t < cumT(3))
        seg_i = int32(3); t0 = cumT(2);
    elseif (maxSeg >= 4) && (T(4) > 0) && (t < cumT(4))
        seg_i = int32(4); t0 = cumT(3);
    else
        seg_i = lastSeg;
        if lastSeg == 1
            t0 = 0.0;
        else
            t0 = cumT(double(lastSeg-1));
        end
        t = cumT(double(lastSeg)); % clamp
        done = true;
    end
end

% ===== 현재 세그먼트 double로 변환해 출력용 저장 =====
seg = double(seg_i);

% ===== 세그먼트 상대시간 =====
tau = t - t0;

% ===== Horner 평가 =====
for d = 1:double(nDOF)
    a5 = coeffs(d,1,seg_i);
    a4 = coeffs(d,2,seg_i);
    a3 = coeffs(d,3,seg_i);
    a2 = coeffs(d,4,seg_i);
    a1 = coeffs(d,5,seg_i);
    a0 = coeffs(d,6,seg_i);
    y(d)    = ((((a5*tau + a4)*tau + a3)*tau + a2)*tau + a1)*tau + a0;
    ydot(d) = ((((5*a5*tau + 4*a4)*tau + 3*a3)*tau + 2*a2)*tau + a1);
end
ydot(4:6) = deg2rad(ydot(4:6));
%y(3) = 0;
%ydot(3) = 0;
end

== matlab function concept3_simulink_RL/Plant/MATLAB Function ==
  data: Docked input; u input; EE output
function EE  = fcn(Docked, u)
EE = true;

if Docked
    EE = false;

end

== matlab function concept3_simulink_RL/QP1/MATLAB Function5 ==
  data: u input; y output; w_prev input; w_new output
function [y, w_new] = fcn(u, w_prev)
% ----------------------------------------------------------
% u      : RL이 출력한 변화율 (Δw)
% w_prev : 이전 step의 가중치 벡터
% y      : 현재 step에서의 출력 w (클리핑된)
% w_new  : 내부 상태 업데이트 값 (다음 스텝에 피드백)
% ----------------------------------------------------------

persistent firstCall
if isempty(firstCall)
    firstCall = true;
end

dt = 1;
sigma = 0.2;
w_max = 1;
w_min = 0;

% --- 1) 첫 스텝에서는 초기 w = sigma*u ---
if firstCall
    w =  u;
    firstCall = false;
else
    % --- 2) 일반 스텝에서는 누적 적분 ---
    w = w_prev + sigma * dt * u;
end

% --- 3) 양방향 포화 (0~1 사이로 제한) ---
w = min(max(w, w_min), w_max);

% --- 4) 출력 ---
y = w;
w_new = w;
end

== matlab function concept3_simulink_RL/QP/Path-Planning /MATLAB Function1 ==
  settings: updateMethod=DISCRETE  sampleTime=0.01
  data: ydot output; y output; clock input; docked input
function [ydot, y] = Poly_traj_homing(clock, docked)
%#codegen

% ── 웨이포인트만 여기서 수정 ──────────────────────────
%      x      y       z    roll  pitch  yaw
WP = [-0.4   1.305   0     90    0      0;    % WP1 (시작)
      -0.4   1.8     0     90    0      0;    % WP2
       2.8   1.8     0     90    0      0;    % WP5
       2.8  -0.2     0.5   90    0     -90];   % WP6 (끝)

T_seg = [20, 40, 30];   % 각 구간 시간 [s]
% ──────────────────────────────────────────────────────

persistent coeffs t_dock
if isempty(coeffs)
    N = length(T_seg);
    coeffs = zeros(6, 6, N);
    for s = 1:N
        T = T_seg(s);
        for d = 1:6
            dy = WP(s+1,d) - WP(s,d);
            coeffs(d,:,s) = [6*dy/T^5, -15*dy/T^4, 10*dy/T^3, 0, 0, WP(s,d)];
        end
    end
end
if isempty(t_dock); t_dock = -1.0; end

y    = zeros(6, 1, 'like', clock);
ydot = zeros(6, 1, 'like', clock);

if ~docked
    y = coeffs(:, 6, 1);
    return;
end
if t_dock < 0; t_dock = clock; end

t    = clock - t_dock;
cumT = cumsum(T_seg);
N    = length(T_seg);

% 구간 선택 — N 구간 자동 대응
seg_i = int32(N);
t0    = cumT(max(N-1, 1));
for s = 1:N
    if t < cumT(s)
        seg_i = int32(s);
        if s == 1;  t0 = 0.0;
        else;       t0 = cumT(s-1);
        end
        break;
    end
end
if t >= cumT(N);  t = cumT(N);  end   % 마지막 구간 끝 클램핑

tau = t - t0;
for d = 1:6
    a5=coeffs(d,1,seg_i); a4=coeffs(d,2,seg_i); a3=coeffs(d,3,seg_i);
    a2=coeffs(d,4,seg_i); a1=coeffs(d,5,seg_i); a0=coeffs(d,6,seg_i);
    y(d)    = ((((a5*tau+a4)*tau+a3)*tau+a2)*tau+a1)*tau+a0;
    ydot(d) = (((5*a5*tau+4*a4)*tau+3*a3)*tau+2*a2)*tau+a1;
end
ydot(4:6) = deg2rad(ydot(4:6));
end

== matlab function concept3_simulink_RL/QP/Subsystem1/Quat2RPY ==
  data: q_current input; RPY output
function RPY = fcn(q_current)

sequence = 'ZYX';

eul_angles_rad_out = quat2eul(q_current', sequence);

eul_angles_deg_out = rad2deg(eul_angles_rad_out);

yaw_deg_out = eul_angles_deg_out(1);
pitch_deg_out = eul_angles_deg_out(2);
roll_deg_out = eul_angles_deg_out(3);

RPY = [roll_deg_out; pitch_deg_out; yaw_deg_out];

== matlab function concept3_simulink_RL/QP1/weight update return ==
  data: u input; w_out output; state_prev input; state_new output
function [w_out, state_new] = weight_update_general(u, state_prev)
% ----------------------------------------------------------
% [w_out, state_new] = weight_update_general(u, state_prev)
%
% u          : RL 액션 벡터 ([-1,1] 범위, 4x1)
% state_prev : 이전 스텝의 가중치 상태 (4x1)
%
% w_out      : 현재 스텝의 가중치 ([-1,1])
% state_new  : 다음 스텝으로 넘길 내부 상태
% ----------------------------------------------------------

persistent firstCall
if isempty(firstCall)
    firstCall = true;
end

% === 파라미터 ===
beta = 0.08;         % EMA smoothing 계수 (0~1)
w_min = -1.0;        % 하한
w_max =  1.0;        % 상한

% === 1) 입력 보정 및 정규화 ===
u = max(min(u(:), 1.0), -1.0);   % [-1,1] 범위 clip

% === 2) 첫 호출 시 ===
if firstCall
    w_f = u;                     % 그대로 반영
    firstCall = false;
else
    % === 3) EMA 스무딩 ===
    w_prev = state_prev(:);
    w_f = (1 - beta) .* w_prev + beta .* u;  % 각 요소별 EMA
end

% === 4) 출력 제한 ===
w_out = min(max(w_f, w_min), w_max);

% === 5) 상태 업데이트 ===
state_new = w_out;
end

== matlab function concept3_simulink_RL/QP1/weight update1 ==
  data: u input; w_out output; state_prev input; state_new output
function [w_out, state_new] = weight_update_general(u, state_prev)
persistent firstCall 
if isempty(firstCall) 
    firstCall = true; 
end 
% 0~1 까지 가는 것에 대해 부드럽게 해주는 시스템
% === 파라미터 === 
 
beta = 0.5; 
% EMA smoothing 계수 (0~1) 
w_min = 0.0; % 하한 
w_max = 1.0; % 상한 

% === 1) 액션 정규화: [-1,1] → [0,1] === 
%u_norm = (u + 1) / 2; 
u_norm = 1*u;
u_norm = min(max(u_norm, w_min), w_max); % clip 
%w_out = u_norm;


% === 2) 첫 스텝이면 바로 반영 === 
% 
 
if firstCall 
    w_f = u_norm; 
    firstCall = false; 
else 
    
    % === 3) EMA 스무딩 === 
    % 
w_prev = state_prev(:); % column 보장 %
%w_f = u_norm; 
w_f = (1 - beta) * w_prev + beta * u_norm(:); 

end 
% === 4) 출력 제한 === 
w_out = min(max(w_f, w_min), w_max); 

% === 5) 상태 업데이트 === 
% 
state_new = w_out; end

== matlab function concept3_simulink_RL/R2L/obs1 ==
  data: q input; y output; qdot input; w_base input; Tau input
function y  = obs(q, qdot, w_base, Tau)
%% --------------------------------------------------------------
% q : [quat_base(4); basepos(3); joint(7)]  (14x1)
% qdot : (7x1)
% H_obs : RL_obs 벡터 (26x1)
% muRL, sigmaRL : 이전 호출의 통계량 (26x1)
% --------------------------------------------------------------
eps = 1e-8;
beta = 0.05;

%% (1) 입력 분리
qbase = q(1:4);
q_joint = q(8:14);

%% (2) 관절 각도/속도 정규화
q_min = [-1.3 -2.9 2.2 -2.8 1.1 1.3 0.1]';
q_max = [2.2 -1.6 4.4 -1.5 3.9 4.4 2.1]';
qdot_max = [0.2 0.07 0.1 0.08 0.23 0.1 0.08]';

q_mid = 0.5 * (q_max + q_min);
q_norm = 2 * (q_joint - q_mid) ./ (q_max - q_min);
qdot_norm = qdot ./ (qdot_max + eps);
qdot_norm = max(min(qdot_norm, 1), -1);

%% (3) 베이스 쿼터니언 정규화
q_base = qbase / (norm(qbase) + eps);   % 정규화
if q_base(1) < 0, q_base = -q_base; end % 연속성 확보

q_ref = [1;0;0;0];                      % 목표자세
q_err = quatmultiply(q_ref.', quatconj(q_base.')).';  % [w x y z]

if q_err(1) < 0, q_err = -q_err; end    % 부호 연속성

att_err_vec = 2 * q_err(2:4);
qbase = att_err_vec / deg2rad(20);   % 약 [-1,1] 범위로 정규화


%% 베이스 속도 정규화
qb_max = 0.004; qb_min = -0.004;
qb_mid = 0.5 * (qb_max + qb_min);
qb_norm = 2 * (w_base - qb_mid) ./ (qb_max - qb_min);

%% 토크 정규화
t_max = 3; t_min = -3;
t_mid = 0.5 * (t_max + t_min);
t_norm = 2 * (Tau - t_mid) ./ (t_max - t_min);

%% (5) 출력 구성

%y = [q_norm; qdot_norm; qbase; qb_norm; t_norm; RL_norm];
y = [q_norm; qdot_norm; qbase; qb_norm; t_norm];
%y = [q_norm; qdot_norm; t_norm];
end

== matlab function concept3_simulink_RL/QP/MATLAB Function ==
  settings: updateMethod=DISCRETE  sampleTime=Tq
  data: alpha input; t input; alpha_s output
function alpha_s = fcn(alpha, t)

alpha_s = alpha_interp(alpha, t);

== matlab function concept3_simulink_RL/QP/Subsystem1/CLIK_fn ==
  data: xcmd input; xdot_cmd output; ee_p input; EE_quat input; pos_err output
function [xdot_cmd, pos_err] = clik(xcmd, ee_p, EE_quat)
Kpos = 5;
Krot = 2;
pos_err = xcmd(1:3) - ee_p;
q_rpy_deg = xcmd(4:6);
q_target = eul2quat([deg2rad(q_rpy_deg(3)),deg2rad(q_rpy_deg(2)),deg2rad(q_rpy_deg(1))], 'ZYX');
q_cur = EE_quat(:)';
if dot(q_target, q_cur) < 0
    q_cur = -q_cur;
end
qc = [q_cur(1), -q_cur(2), -q_cur(3), -q_cur(4)];
w1=q_target(1); x1=q_target(2); yt=q_target(3); z1=q_target(4);
w2=qc(1); x2=qc(2); y2=qc(3); z2=qc(4);
e_rot = [w1*x2+x1*w2+yt*z2-z1*y2; w1*y2-x1*z2+yt*w2+z1*x2; w1*z2+x1*y2-yt*x2+z1*w2];
v_cmd = min(max(Kpos*pos_err, -0.2), 0.2);
w_cmd = min(max(Krot*e_rot, -0.09), 0.09);
xdot_cmd = [w_cmd; v_cmd];

== matlab function concept3_simulink_RL/RL/MATLAB Function ==
  data: u input; y output
function y = fcn(u)

y = double(u);

== matlab function concept3_simulink_RL/RL/MATLAB Function1 ==
  data: u input; obs output
function obs = fcn(u)

obs = RL_obs(u);

== matlab function concept3_simulink_RL/RL/MATLAB Function2 ==
  data: r_tot output; u input; r output
function [r_tot, r] = fcn(u)


[r_tot, r] = RL_r2(u);

== matlab function concept3_simulink_RL/QP/Path-Planning /MATLAB Function2 ==
  settings: updateMethod=DISCRETE  sampleTime=0.01
  data: ydot output; y output; clock input; docked input
function [ydot, y] = Poly_traj_homing(clock, docked)
%#codegen

T1=10; T2=25; T3=20; T4=25; T5=30;

coeffs = zeros(6, 6, 5, 'like', clock);

% Segment 1 (10s): WP1→WP2, Δy=0.195
coeffs(:,:,1) = [ ...
 0           0            0           0  0  -0.4;
 1.17e-5    -2.925e-4     1.95e-3     0  0   1.305;
 0           0            0           0  0   0;
 0           0            0           0  0   90;
 0           0            0           0  0   0;
 0           0            0           0  0   0];

% Segment 2 (25s): WP2→WP3, z=0 고정
coeffs(:,:,2) = [ ...
 0          0          0          0  0  -0.4;
 0          0          0          0  0   1.5;
 0          0          0          0  0   0;    % ← 전체 0으로
 0          0          0          0  0   90;
 0          0          0          0  0   0;
 0          0          0          0  0   0];


% Segment 3 (20s): WP3→WP4, Δx=0.3, Δyaw=90
coeffs(:,:,3) = [ ...
 5.625e-7  -2.8125e-5   3.75e-4   0  0  -0.4;
 0          0           0         0  0   1.5;
 0          0           0         0  0   0.05;
 0          0           0         0  0   90;
 0          0           0         0  0   0;
 1.6875e-4 -8.4375e-3   1.125e-1  0  0   0];

% Segment 4 (25s): WP4→WP5, Δx=2.9
coeffs(:,:,4) = [ ...
 1.78176e-6  -1.1136e-4   1.856e-3  0  0  -0.1;
 0            0           0         0  0   1.5;
 0            0           0         0  0   0.0;
 0            0           0         0  0   90;
 0            0           0         0  0   0;
 0            0           0         0  0   90];

% Segment 5 (30s): WP5→WP6, Δy=-1.7, Δz=0.5
coeffs(:,:,5) = [ ...
 0             0             0            0  0   2.8;
-4.19753e-7    3.14815e-5   -6.29630e-4   0  0   1.5;
 1.23457e-7   -9.25926e-6    1.85185e-4   0  0   0;    % ← z: 0→0.5
 0             0             0            0  0   90;
 0             0             0            0  0   0;
 0             0             0            0  0   90];

y    = zeros(6, 1, 'like', clock);
ydot = zeros(6, 1, 'like', clock);

persistent t_dock
if isempty(t_dock)
    t_dock = -1.0;
end

if ~docked
    y = coeffs(:, 6, 1);
    return;
end

if t_dock < 0
    t_dock = clock;
end

t = clock - t_dock;

cumT = [T1, T1+T2, T1+T2+T3, T1+T2+T3+T4, T1+T2+T3+T4+T5];

if t <= 0
    seg_i = int32(1); t0 = 0.0;
elseif t < cumT(1)
    seg_i = int32(1); t0 = 0.0;
elseif t < cumT(2)
    seg_i = int32(2); t0 = cumT(1);
elseif t < cumT(3)
    seg_i = int32(3); t0 = cumT(2);
elseif t < cumT(4)
    seg_i = int32(4); t0 = cumT(3);
elseif t < cumT(5)
    seg_i = int32(5); t0 = cumT(4);
else
    seg_i = int32(5); t0 = cumT(4);
    t = cumT(5);
end

tau = t - t0;

for d = 1:6
    a5 = coeffs(d,1,seg_i); a4 = coeffs(d,2,seg_i); a3 = coeffs(d,3,seg_i);
    a2 = coeffs(d,4,seg_i); a1 = coeffs(d,5,seg_i); a0 = coeffs(d,6,seg_i);
    y(d)    = ((((a5*tau + a4)*tau + a3)*tau + a2)*tau + a1)*tau + a0;
    ydot(d) = (((5*a5*tau + 4*a4)*tau + 3*a3)*tau + 2*a2)*tau + a1;
end
ydot(4:6) = deg2rad(ydot(4:6));
end

== matlab function concept3_simulink_RL/R2L/MATLAB Function2 ==
  data: q input; y output; qdot input; w_base input; Tau input
function y = obs(q, qdot, w_base, Tau)
    % 1. 외부 함수로 인식시키기 위해 coder.extrinsic 선언 (매우 중요)
    coder.extrinsic('obs');
    
    % 2. 출력 변수 'y'의 크기와 데이터 타입을 미리 명시 (Pre-allocation)
    % Simulink는 컴파일 시점에 출력 크기를 알아야 하므로 이 과정이 필수입니다.
    % 7(q) + 7(qdot) + 3(qbase) + 3(w_base) + 7(Tau) = 27 (크기 확인 필요)
    y = zeros(27, 1); 
    
    % 3. 외부 스크립트(obs_ext.m) 호출
    y = obs(q, qdot, w_base, Tau);
end

== matlab function concept3_simulink_RL/QP/Path-Planning /MATLAB Function3 ==
  data: ydot output; y output; clock input
function [ydot, y] = Poly_traj_610(clock)
%#codegen

T1 = 32.8718048721934;
T2 = 58.000;
T3 = 20.0;
T4 = 26.9258240356725;
T5 = 10;
T  = [T1, T2, T3, T4, T5];

coeffs = zeros(6, 6, 5, 'like', clock);

% Segment 1: (2.5,0.35,0) → (2.5,1.2,0.5), yaw=-90° 유지
coeffs(:,:,1) = [ ...
 0                   -0                    0                    0  0   2.5;
 1.32877798661e-07   -1.09198326736e-05    0.000239303072589    0  0   0.35;
 7.81634109771e-08   -6.42343098446e-06    0.000140766513288    0  0   0;
 0                   -0                    0                    0  0  -90;
 0                   -0                    0                    0  0   0;
 0                   -0                    0                    0  0  -90];

% Segment 2: x 이동 2.5→-0.4, y/z=(1.2,0.5) 고정
coeffs(:,:,2) = [ ...
-2.65099726983e-08    3.84394604125e-06   -0.000148632580262    0  0   2.5;
 0                   -0                    0                    0  0   1.2;
 0                   -0                    0                    0  0   0.5;
 0                   -0                    0                    0  0  -90;
 0                   -0                    0                    0  0   0;
 0                   -0                    0                    0  0  -90];

% Segment 3: 위치 고정, yaw -90°→0° 회전
coeffs(:,:,3) = [ ...
 0                   -0                    0                    0  0  -0.4;
 0                   -0                    0                    0  0   1.2;
 0                   -0                    0                    0  0   0.5;
 0                   -0                    0                    0  0  -90;
 0                   -0                    0                    0  0   0;
 0.00016875          -0.0084375            0.1125               0  0  -90];

% Segment 4: y:1.2→0, z:0.5→0
coeffs(:,:,4) = [ ...
 0                   -0                    0                    0  0  -0.4;
-8.47883589298e-08    5.70749108205e-06   -0.000102452600374    0  0   1.2;
-2.11970897325e-07    1.42687277051e-05   -0.000256131500934    0  0   0.5;
 0                   -0                    0                    0  0  -90;
 0                   -0                    0                    0  0   0;
 0                   -0                    0                    0  0   0];

% Segment 5: (-0.4,1,0) → (-0.4,0.8,0), 자세 유지 (yaw=0°)

coeffs(:,:,5) = [ ...
 0         0        0        0  0  -0.4;
-1.2e-05   3.0e-04 -2.0e-03  0  0   1.0;
 0         0        0        0  0   0;
 0         0        0        0  0  -90;
 0         0        0        0  0   0;
 0         0        0        0  0   0];

%{
% Segment 5: (-0.4,1,0) → (-0.4,0.795,0), 자세 유지 (yaw=0°)
coeffs(:,:,5) = [ ...
 0          0          0         0  0  -0.4;
-1.23e-05   3.075e-04 -2.05e-03  0  0   1.0;
 0          0          0         0  0   0;
 0          0          0         0  0  -90;
 0          0          0         0  0   0;
 0          0          0         0  0   0];
%}

y    = zeros(6, 1, 'like', clock);
ydot = zeros(6, 1, 'like', clock);
done = false;

cumT = [T(1), T(1)+T(2), T(1)+T(2)+T(3), T(1)+T(2)+T(3)+T(4), ...
        T(1)+T(2)+T(3)+T(4)+T(5)];

t = clock;
if t <= 0
    seg_i = int32(1); t0 = 0.0;
elseif t < cumT(1)
    seg_i = int32(1); t0 = 0.0;
elseif t < cumT(2)
    seg_i = int32(2); t0 = cumT(1);
elseif t < cumT(3)
    seg_i = int32(3); t0 = cumT(2);
elseif t < cumT(4)
    seg_i = int32(4); t0 = cumT(3);
elseif t < cumT(5)
    seg_i = int32(5); t0 = cumT(4);
else
    seg_i = int32(5); t0 = cumT(4);   % ← 기존 4에서 5로 변경
    t = cumT(5);                        % ← 기존 cumT(4)에서 cumT(5)로 변경
    done = true;
end

seg = double(seg_i);
tau = t - t0;

for d = 1:6
    a5 = coeffs(d,1,seg_i); a4 = coeffs(d,2,seg_i); a3 = coeffs(d,3,seg_i);
    a2 = coeffs(d,4,seg_i); a1 = coeffs(d,5,seg_i); a0 = coeffs(d,6,seg_i);
    y(d)    = ((((a5*tau + a4)*tau + a3)*tau + a2)*tau + a1)*tau + a0;
    ydot(d) = (((5*a5*tau + 4*a4)*tau + 3*a3)*tau + 2*a2)*tau + a1;
end
ydot(4:6) = deg2rad(ydot(4:6));
end
